simulink library "myLibrary"  (R2023b)
settings: Solver=VariableStepAuto  StartTime=0.0  StopTime=10.0  RelTol=1e-3
undefined symbols (not defined in the file): Cac_n1, ctrl1, Da, Discrete, dtha, ee_sli_rtmsupport, FA, gcbh, Ha, Ini, init_DCline, init_IPC, init_line, init_load, init_SG, init_shunt, init_TH, init_trafo, init_VSC, initMachineBlocks, Ka, Lf, Llkd_pu, Llkq1_pu, magnitude, NET, P, plots_step, q0, Rac_n1, Radd, Rkd_pu, Rkq1_pu, Rload_add, sim_config, sps_rtmsupport, spsSteamTurbineModel, T_DC_NET, T_global, T_IPC, T_load, T_NET, T_SG, T_shunt, T_STATCOM, T_TH, T_trafo, T_VSC, Ts, tstep, Udiff_a, V1
libraries: spsSeriesRLCBranchLib x105, eeGeneralControl x72, $bdroot x70, spsCurrentMeasurementLib x48, spsParallelRLCBranchLib x39, spsVoltageMeasurementLib x33, spsControlledVoltageSourceLib x27, spsFirstOrderFilterLib x16, dspsigops x6, spsThreePhaseVIMeasurementLib x5, spsPLL3phLib x4, spsThreePhaseBreakerLib x3
(part 9 of 12)

== system myLibrary/STATCOM/Control/Rotació ==
  V_q_diff : Inport
  V_d_diff : Inport  Port=2
  V_0_diff : Inport  Port=3
  Angle : Inport  Port=4
  Constant{2,5..7} (4 alike) : Constant  Value=0
  Constant8 : Constant
  Demux : Demux  Outputs=3
  Display : Display
  Gain1 : Gain  Gain=-1
  Matrix Concatenate : Concatenate  NumInputs=3  Mode=Multidimensional array  ConcatenateDimension=2
  Mux{,1..3} (4 alike) : Mux  Inputs=3
  Product : Product  Multiplication=Matrix(*)
  Trigonometric Function : Trigonometry  Operator=cos
  Trigonometric Function1 : Trigonometry
  Trigonometric Function2 : Trigonometry
  Trigonometric Function3 : Trigonometry  Operator=cos
  V_alfa_diff : Outport  VectorParamsAs1DForOutWhenUnconnected=off
  V_beta_diff : Outport  Port=2  VectorParamsAs1DForOutWhenUnconnected=off
  V_0 : Outport  Port=3  VectorParamsAs1DForOutWhenUnconnected=off
  wires:
  Angle/1 -> Trigonometric Function1/1, Trigonometric Function2/1, Trigonometric Function3/1, Trigonometric Function/1
  Trigonometric Function2/1 -> Mux2/1
  Gain1/1 -> Mux1/2
  Trigonometric Function/1 -> Mux1/1
  V_0_diff/1 -> Mux/3
  V_d_diff/1 -> Mux/2
  V_q_diff/1 -> Mux/1
  Matrix Concatenate/1 -> Product/1, Display/1
  Mux/1 -> Product/2
  Demux/3 -> V_0/1
  Demux/2 -> V_beta_diff/1
  Demux/1 -> V_alfa_diff/1
  Product/1 -> Demux/1
  Mux1/1 -> Matrix Concatenate/1
  Mux3/1 -> Matrix Concatenate/3
  Mux2/1 -> Matrix Concatenate/2
  Constant8/1 -> Mux3/3
  Constant7/1 -> Mux3/2
  Constant6/1 -> Mux3/1
  Constant5/1 -> Mux2/3
  Trigonometric Function3/1 -> Mux2/2
  Constant2/1 -> Mux1/3
  Trigonometric Function1/1 -> Gain1/1

== system myLibrary/STATCOM/Control/Subsystem ==
  Uq : Inport
  Ud : Inport  Port=2
  iq : Inport  Port=3
  id : Inport  Port=4
  Gain2 : Gain  Gain=3/2
  Product : Product
  Product1 : Product
  Sum8 : Sum
  Pac : Outport
  wires:
  Uq/1 -> Product/1
  Product/1 -> Sum8/1
  iq/1 -> Product/2
  id/1 -> Product1/2
  Gain2/1 -> Pac/1
  Ud/1 -> Product1/1
  Product1/1 -> Sum8/2
  Sum8/1 -> Gain2/1

== system myLibrary/qd transform/qd0 Transformation/Matriu T ==
  u : Inport
  Constant : Constant  Value=(2/3)*[1/2 1/2 1/2]
  Fcn : Fcn  Expr=(2/3)*cos(u)
  Fcn1 : Fcn  Expr=(2/3)*cos(u-(2*pi)/3)
  Fcn2 : Fcn  Expr=(2/3)*cos(u+(2*pi)/3)
  Fcn3 : Fcn  Expr=(2/3)*sin(u)
  Fcn4 : Fcn  Expr=(2/3)*sin(u-(2*pi)/3)
  Fcn5 : Fcn  Expr=(2/3)*sin(u+(2*pi)/3)
  Math Function : Math  Operator=transpose  SignedPower=on
  Matrix Concatenate : Concatenate  NumInputs=3  Mode=Multidimensional array  ConcatenateDimension=2
  Mux : Mux  Inputs=3
  Mux1 : Mux  Inputs=3
  Out1 : Outport  VectorParamsAs1DForOutWhenUnconnected=off
  wires:
  u/1 -> Fcn/1, Fcn1/1, Fcn2/1, Fcn3/1, Fcn4/1, Fcn5/1
  Fcn3/1 -> Mux1/1
  Fcn4/1 -> Mux1/2
  Fcn5/1 -> Mux1/3
  Mux/1 -> Matrix Concatenate/1
  Constant/1 -> Matrix Concatenate/3
  Fcn/1 -> Mux/1
  Fcn1/1 -> Mux/2
  Fcn2/1 -> Mux/3
  Mux1/1 -> Matrix Concatenate/2
  Matrix Concatenate/1 -> Math Function/1
  Math Function/1 -> Out1/1

== system myLibrary/AC-GFOL_DC-GFOL/Control Pac2/Is/Matriu T ==
  u : Inport
  Constant : Constant  Value=(2/3)*[1/2 1/2 1/2]
  Fcn : Fcn  Expr=(2/3)*cos(u)
  Fcn1 : Fcn  Expr=(2/3)*cos(u-(2*pi)/3)
  Fcn2 : Fcn  Expr=(2/3)*cos(u+(2*pi)/3)
  Fcn3 : Fcn  Expr=(2/3)*sin(u)
  Fcn4 : Fcn  Expr=(2/3)*sin(u-(2*pi)/3)
  Fcn5 : Fcn  Expr=(2/3)*sin(u+(2*pi)/3)
  Math Function : Math  Operator=transpose  SignedPower=on
  Matrix Concatenate : Concatenate  NumInputs=3  Mode=Multidimensional array  ConcatenateDimension=2
  Mux : Mux  Inputs=3
  Mux1 : Mux  Inputs=3
  Out1 : Outport  VectorParamsAs1DForOutWhenUnconnected=off
  wires:
  u/1 -> Fcn/1, Fcn1/1, Fcn2/1, Fcn3/1, Fcn4/1, Fcn5/1
  Fcn3/1 -> Mux1/1
  Fcn4/1 -> Mux1/2
  Fcn5/1 -> Mux1/3
  Mux/1 -> Matrix Concatenate/1
  Constant/1 -> Matrix Concatenate/3
  Fcn/1 -> Mux/1
  Fcn1/1 -> Mux/2
  Fcn2/1 -> Mux/3
  Mux1/1 -> Matrix Concatenate/2
  Matrix Concatenate/1 -> Math Function/1
  Math Function/1 -> Out1/1

== system myLibrary/AC-GFOL_DC-GFOL/Control Pac2/Is2/Matriu T ==
  u : Inport
  Constant : Constant  Value=(2/3)*[1/2 1/2 1/2]
  Fcn : Fcn  Expr=(2/3)*cos(u)
  Fcn1 : Fcn  Expr=(2/3)*cos(u-(2*pi)/3)
  Fcn2 : Fcn  Expr=(2/3)*cos(u+(2*pi)/3)
  Fcn3 : Fcn  Expr=(2/3)*sin(u)
  Fcn4 : Fcn  Expr=(2/3)*sin(u-(2*pi)/3)
  Fcn5 : Fcn  Expr=(2/3)*sin(u+(2*pi)/3)
  Math Function : Math  Operator=transpose  SignedPower=on
  Matrix Concatenate : Concatenate  NumInputs=3  Mode=Multidimensional array  ConcatenateDimension=2
  Mux : Mux  Inputs=3
  Mux1 : Mux  Inputs=3
  Out1 : Outport  VectorParamsAs1DForOutWhenUnconnected=off
  wires:
  u/1 -> Fcn/1, Fcn1/1, Fcn2/1, Fcn3/1, Fcn4/1, Fcn5/1
  Fcn3/1 -> Mux1/1
  Fcn4/1 -> Mux1/2
  Fcn5/1 -> Mux1/3
  Mux/1 -> Matrix Concatenate/1
  Constant/1 -> Matrix Concatenate/3
  Fcn/1 -> Mux/1
  Fcn1/1 -> Mux/2
  Fcn2/1 -> Mux/3
  Mux1/1 -> Matrix Concatenate/2
  Matrix Concatenate/1 -> Math Function/1
  Math Function/1 -> Out1/1

== system myLibrary/AC-GFOL_DC-GFOL/Control Pac2/l_DC_alfa//beta/Clarke ==
  Isum : Inport
  Constant : Constant
  Constant1 : Constant  Value=-1/2
  Constant2 : Constant  Value=-1/2
  Constant3 : Constant  Value=0
  Constant4 : Constant  Value=-sqrt(3)/2
  Constant5 : Constant  Value=sqrt(3)/2
  Constant6 : Constant  Value=1/2
  Constant7 : Constant  Value=1/2
  Constant8 : Constant  Value=1/2
  Demux : Demux  Outputs=3
  Display : Display
  Gain : Gain  Gain=2/3
  Math Function : Math  Operator=transpose  SignedPower=on
  Matrix Concatenate : Concatenate  NumInputs=3  Mode=Multidimensional array  ConcatenateDimension=2
  Mux1 : Mux  Inputs=3
  Mux2 : Mux  Inputs=3
  Mux3 : Mux  Inputs=3
  Product : Product  Multiplication=Matrix(*)
  I_alfa : Outport  VectorParamsAs1DForOutWhenUnconnected=off
  I_beta : Outport  Port=2  VectorParamsAs1DForOutWhenUnconnected=off
  I_0 : Outport  Port=3  VectorParamsAs1DForOutWhenUnconnected=off
  wires:
  Constant/1 -> Mux1/1
  Constant1/1 -> Mux1/2
  Constant2/1 -> Mux1/3
  Constant3/1 -> Mux2/1
  Constant4/1 -> Mux2/2
  Constant5/1 -> Mux2/3
  Constant6/1 -> Mux3/1
  Constant7/1 -> Mux3/2
  Constant8/1 -> Mux3/3
  Math Function/1 -> Gain/1
  Matrix Concatenate/1 -> Math Function/1
  Mux2/1 -> Matrix Concatenate/2
  Mux3/1 -> Matrix Concatenate/3
  Mux1/1 -> Matrix Concatenate/1
  Product/1 -> Demux/1
  Demux/1 -> I_alfa/1
  Demux/2 -> I_beta/1
  Demux/3 -> I_0/1
  Gain/1 -> Display/1, Product/1
  Isum/1 -> Product/2

== system myLibrary/AC-GFOL_DC-GFOR/Control Pac2/Is/Matriu T ==
  u : Inport
  Constant : Constant  Value=(2/3)*[1/2 1/2 1/2]
  Fcn : Fcn  Expr=(2/3)*cos(u)
  Fcn1 : Fcn  Expr=(2/3)*cos(u-(2*pi)/3)
  Fcn2 : Fcn  Expr=(2/3)*cos(u+(2*pi)/3)
  Fcn3 : Fcn  Expr=(2/3)*sin(u)
  Fcn4 : Fcn  Expr=(2/3)*sin(u-(2*pi)/3)
  Fcn5 : Fcn  Expr=(2/3)*sin(u+(2*pi)/3)
  Math Function : Math  Operator=transpose  SignedPower=on
  Matrix Concatenate : Concatenate  NumInputs=3  Mode=Multidimensional array  ConcatenateDimension=2
  Mux : Mux  Inputs=3
  Mux1 : Mux  Inputs=3
  Out1 : Outport  VectorParamsAs1DForOutWhenUnconnected=off
  wires:
  u/1 -> Fcn/1, Fcn1/1, Fcn2/1, Fcn3/1, Fcn4/1, Fcn5/1
  Fcn3/1 -> Mux1/1
  Fcn4/1 -> Mux1/2
  Fcn5/1 -> Mux1/3
  Mux/1 -> Matrix Concatenate/1
  Constant/1 -> Matrix Concatenate/3
  Fcn/1 -> Mux/1
  Fcn1/1 -> Mux/2
  Fcn2/1 -> Mux/3
  Mux1/1 -> Matrix Concatenate/2
  Matrix Concatenate/1 -> Math Function/1
  Math Function/1 -> Out1/1

== system myLibrary/AC-GFOL_DC-GFOR/Control Pac2/Is2/Matriu T ==
  u : Inport
  Constant : Constant  Value=(2/3)*[1/2 1/2 1/2]
  Fcn : Fcn  Expr=(2/3)*cos(u)
  Fcn1 : Fcn  Expr=(2/3)*cos(u-(2*pi)/3)
  Fcn2 : Fcn  Expr=(2/3)*cos(u+(2*pi)/3)
  Fcn3 : Fcn  Expr=(2/3)*sin(u)
  Fcn4 : Fcn  Expr=(2/3)*sin(u-(2*pi)/3)
  Fcn5 : Fcn  Expr=(2/3)*sin(u+(2*pi)/3)
  Math Function : Math  Operator=transpose  SignedPower=on
  Matrix Concatenate : Concatenate  NumInputs=3  Mode=Multidimensional array  ConcatenateDimension=2
  Mux : Mux  Inputs=3
  Mux1 : Mux  Inputs=3
  Out1 : Outport  VectorParamsAs1DForOutWhenUnconnected=off
  wires:
  u/1 -> Fcn/1, Fcn1/1, Fcn2/1, Fcn3/1, Fcn4/1, Fcn5/1
  Fcn3/1 -> Mux1/1
  Fcn4/1 -> Mux1/2
  Fcn5/1 -> Mux1/3
  Mux/1 -> Matrix Concatenate/1
  Constant/1 -> Matrix Concatenate/3
  Fcn/1 -> Mux/1
  Fcn1/1 -> Mux/2
  Fcn2/1 -> Mux/3
  Mux1/1 -> Matrix Concatenate/2
  Matrix Concatenate/1 -> Math Function/1
  Math Function/1 -> Out1/1

== system myLibrary/AC-GFOL_DC-GFOR/Control Pac2/l_DC_alfa//beta/Clarke ==
  Isum : Inport
  Constant : Constant
  Constant1 : Constant  Value=-1/2
  Constant2 : Constant  Value=-1/2
  Constant3 : Constant  Value=0
  Constant4 : Constant  Value=-sqrt(3)/2
  Constant5 : Constant  Value=sqrt(3)/2
  Constant6 : Constant  Value=1/2
  Constant7 : Constant  Value=1/2
  Constant8 : Constant  Value=1/2
  Demux : Demux  Outputs=3
  Display : Display
  Gain : Gain  Gain=2/3
  Math Function : Math  Operator=transpose  SignedPower=on
  Matrix Concatenate : Concatenate  NumInputs=3  Mode=Multidimensional array  ConcatenateDimension=2
  Mux1 : Mux  Inputs=3
  Mux2 : Mux  Inputs=3
  Mux3 : Mux  Inputs=3
  Product : Product  Multiplication=Matrix(*)
  I_alfa : Outport  VectorParamsAs1DForOutWhenUnconnected=off
  I_beta : Outport  Port=2  VectorParamsAs1DForOutWhenUnconnected=off
  I_0 : Outport  Port=3  VectorParamsAs1DForOutWhenUnconnected=off
  wires:
  Constant/1 -> Mux1/1
  Constant1/1 -> Mux1/2
  Constant2/1 -> Mux1/3
  Constant3/1 -> Mux2/1
  Constant4/1 -> Mux2/2
  Constant5/1 -> Mux2/3
  Constant6/1 -> Mux3/1
  Constant7/1 -> Mux3/2
  Constant8/1 -> Mux3/3
  Math Function/1 -> Gain/1
  Matrix Concatenate/1 -> Math Function/1
  Mux2/1 -> Matrix Concatenate/2
  Mux3/1 -> Matrix Concatenate/3
  Mux1/1 -> Matrix Concatenate/1
  Product/1 -> Demux/1
  Demux/1 -> I_alfa/1
  Demux/2 -> I_beta/1
  Demux/3 -> I_0/1
  Gain/1 -> Display/1, Product/1
  Isum/1 -> Product/2

== system myLibrary/AC-GFOR_DC-GFOL/Control Pac2/Is/Matriu T ==
  u : Inport
  Constant : Constant  Value=(2/3)*[1/2 1/2 1/2]
  Fcn : Fcn  Expr=(2/3)*cos(u)
  Fcn1 : Fcn  Expr=(2/3)*cos(u-(2*pi)/3)
  Fcn2 : Fcn  Expr=(2/3)*cos(u+(2*pi)/3)
  Fcn3 : Fcn  Expr=(2/3)*sin(u)
  Fcn4 : Fcn  Expr=(2/3)*sin(u-(2*pi)/3)
  Fcn5 : Fcn  Expr=(2/3)*sin(u+(2*pi)/3)
  Math Function : Math  Operator=transpose  SignedPower=on
  Matrix Concatenate : Concatenate  NumInputs=3  Mode=Multidimensional array  ConcatenateDimension=2
  Mux : Mux  Inputs=3
  Mux1 : Mux  Inputs=3
  Out1 : Outport  VectorParamsAs1DForOutWhenUnconnected=off
  wires:
  Math Function/1 -> Out1/1
  Matrix Concatenate/1 -> Math Function/1
  Mux1/1 -> Matrix Concatenate/2
  Fcn2/1 -> Mux/3
  Fcn1/1 -> Mux/2
  Fcn/1 -> Mux/1
  Constant/1 -> Matrix Concatenate/3
  Mux/1 -> Matrix Concatenate/1
  Fcn5/1 -> Mux1/3
  Fcn4/1 -> Mux1/2
  Fcn3/1 -> Mux1/1
  u/1 -> Fcn5/1, Fcn4/1, Fcn3/1, Fcn2/1, Fcn1/1, Fcn/1

== system myLibrary/AC-GFOR_DC-GFOL/Control Pac2/Is2/Matriu T ==
  u : Inport
  Constant : Constant  Value=(2/3)*[1/2 1/2 1/2]
  Fcn : Fcn  Expr=(2/3)*cos(u)
  Fcn1 : Fcn  Expr=(2/3)*cos(u-(2*pi)/3)
  Fcn2 : Fcn  Expr=(2/3)*cos(u+(2*pi)/3)
  Fcn3 : Fcn  Expr=(2/3)*sin(u)
  Fcn4 : Fcn  Expr=(2/3)*sin(u-(2*pi)/3)
  Fcn5 : Fcn  Expr=(2/3)*sin(u+(2*pi)/3)
  Math Function : Math  Operator=transpose  SignedPower=on
  Matrix Concatenate : Concatenate  NumInputs=3  Mode=Multidimensional array  ConcatenateDimension=2
  Mux : Mux  Inputs=3
  Mux1 : Mux  Inputs=3
  Out1 : Outport  VectorParamsAs1DForOutWhenUnconnected=off
  wires:
  Math Function/1 -> Out1/1
  Matrix Concatenate/1 -> Math Function/1
  Mux1/1 -> Matrix Concatenate/2
  Fcn2/1 -> Mux/3
  Fcn1/1 -> Mux/2
  Fcn/1 -> Mux/1
  Constant/1 -> Matrix Concatenate/3
  Mux/1 -> Matrix Concatenate/1
  Fcn5/1 -> Mux1/3
  Fcn4/1 -> Mux1/2
  Fcn3/1 -> Mux1/1
  u/1 -> Fcn5/1, Fcn4/1, Fcn3/1, Fcn2/1, Fcn1/1, Fcn/1

== system myLibrary/AC-GFOR_DC-GFOL/Control Pac2/l_DC_alfa//beta/Clarke ==
  Isum : Inport
  Constant : Constant
  Constant1 : Constant  Value=-1/2
  Constant2 : Constant  Value=-1/2
  Constant3 : Constant  Value=0
  Constant4 : Constant  Value=-sqrt(3)/2
  Constant5 : Constant  Value=sqrt(3)/2
  Constant6 : Constant  Value=1/2
  Constant7 : Constant  Value=1/2
  Constant8 : Constant  Value=1/2
  Demux : Demux  Outputs=3
  Display : Display
  Gain : Gain  Gain=2/3
  Math Function : Math  Operator=transpose  SignedPower=on
  Matrix Concatenate : Concatenate  NumInputs=3  Mode=Multidimensional array  ConcatenateDimension=2
  Mux1 : Mux  Inputs=3
  Mux2 : Mux  Inputs=3
  Mux3 : Mux  Inputs=3
  Product : Product  Multiplication=Matrix(*)
  I_alfa : Outport  VectorParamsAs1DForOutWhenUnconnected=off
  I_beta : Outport  Port=2  VectorParamsAs1DForOutWhenUnconnected=off
  I_0 : Outport  Port=3  VectorParamsAs1DForOutWhenUnconnected=off
  wires:
  Isum/1 -> Product/2
  Gain/1 -> Product/1, Display/1
  Demux/3 -> I_0/1
  Demux/2 -> I_beta/1
  Demux/1 -> I_alfa/1
  Product/1 -> Demux/1
  Mux1/1 -> Matrix Concatenate/1
  Mux3/1 -> Matrix Concatenate/3
  Mux2/1 -> Matrix Concatenate/2
  Matrix Concatenate/1 -> Math Function/1
  Math Function/1 -> Gain/1
  Constant8/1 -> Mux3/3
  Constant7/1 -> Mux3/2
  Constant6/1 -> Mux3/1
  Constant5/1 -> Mux2/3
  Constant4/1 -> Mux2/2
  Constant3/1 -> Mux2/1
  Constant2/1 -> Mux1/3
  Constant1/1 -> Mux1/2
  Constant/1 -> Mux1/1

== system myLibrary/GFOL/Control/Is/Matriu T ==
  u : Inport
  Constant : Constant  Value=(2/3)*[1/2 1/2 1/2]
  Fcn : Fcn  Expr=(2/3)*cos(u)
  Fcn1 : Fcn  Expr=(2/3)*cos(u-(2*pi)/3)
  Fcn2 : Fcn  Expr=(2/3)*cos(u+(2*pi)/3)
  Fcn3 : Fcn  Expr=(2/3)*sin(u)
  Fcn4 : Fcn  Expr=(2/3)*sin(u-(2*pi)/3)
  Fcn5 : Fcn  Expr=(2/3)*sin(u+(2*pi)/3)
  Math Function : Math  Operator=transpose  SignedPower=on
  Matrix Concatenate : Concatenate  NumInputs=3  Mode=Multidimensional array  ConcatenateDimension=2
  Mux : Mux  Inputs=3
  Mux1 : Mux  Inputs=3
  Out1 : Outport  VectorParamsAs1DForOutWhenUnconnected=off
  wires:
  u/1 -> Fcn/1, Fcn1/1, Fcn2/1, Fcn3/1, Fcn4/1, Fcn5/1
  Fcn3/1 -> Mux1/1
  Fcn4/1 -> Mux1/2
  Fcn5/1 -> Mux1/3
  Mux/1 -> Matrix Concatenate/1
  Constant/1 -> Matrix Concatenate/3
  Fcn/1 -> Mux/1
  Fcn1/1 -> Mux/2
  Fcn2/1 -> Mux/3
  Mux1/1 -> Matrix Concatenate/2
  Matrix Concatenate/1 -> Math Function/1
  Math Function/1 -> Out1/1

== system myLibrary/GFOL/Control/Is1/Matriu T ==
  u : Inport
  Constant : Constant  Value=(2/3)*[1/2 1/2 1/2]
  Fcn : Fcn  Expr=(2/3)*cos(u)
  Fcn1 : Fcn  Expr=(2/3)*cos(u-(2*pi)/3)
  Fcn2 : Fcn  Expr=(2/3)*cos(u+(2*pi)/3)
  Fcn3 : Fcn  Expr=(2/3)*sin(u)
  Fcn4 : Fcn  Expr=(2/3)*sin(u-(2*pi)/3)
  Fcn5 : Fcn  Expr=(2/3)*sin(u+(2*pi)/3)
  Math Function : Math  Operator=transpose  SignedPower=on
  Matrix Concatenate : Concatenate  NumInputs=3  Mode=Multidimensional array  ConcatenateDimension=2
  Mux : Mux  Inputs=3
  Mux1 : Mux  Inputs=3
  Out1 : Outport  VectorParamsAs1DForOutWhenUnconnected=off
  wires:
  Math Function/1 -> Out1/1
  Matrix Concatenate/1 -> Math Function/1
  Mux1/1 -> Matrix Concatenate/2
  Fcn2/1 -> Mux/3
  Fcn1/1 -> Mux/2
  Fcn/1 -> Mux/1
  Constant/1 -> Matrix Concatenate/3
  Mux/1 -> Matrix Concatenate/1
  Fcn5/1 -> Mux1/3
  Fcn4/1 -> Mux1/2
  Fcn3/1 -> Mux1/1
  u/1 -> Fcn5/1, Fcn4/1, Fcn3/1, Fcn2/1, Fcn1/1, Fcn/1

== system myLibrary/GFOL/Control/Is3/Matriu T ==
  u : Inport
  Constant : Constant  Value=(2/3)*[1/2 1/2 1/2]
  Fcn : Fcn  Expr=(2/3)*cos(u)
  Fcn1 : Fcn  Expr=(2/3)*cos(u-(2*pi)/3)
  Fcn2 : Fcn  Expr=(2/3)*cos(u+(2*pi)/3)
  Fcn3 : Fcn  Expr=(2/3)*sin(u)
  Fcn4 : Fcn  Expr=(2/3)*sin(u-(2*pi)/3)
  Fcn5 : Fcn  Expr=(2/3)*sin(u+(2*pi)/3)
  Math Function : Math  Operator=transpose  SignedPower=on
  Matrix Concatenate : Concatenate  NumInputs=3  Mode=Multidimensional array  ConcatenateDimension=2
  Mux : Mux  Inputs=3
  Mux1 : Mux  Inputs=3
  Out1 : Outport  VectorParamsAs1DForOutWhenUnconnected=off
  wires:
  u/1 -> Fcn/1, Fcn1/1, Fcn2/1, Fcn3/1, Fcn4/1, Fcn5/1
  Fcn3/1 -> Mux1/1
  Fcn4/1 -> Mux1/2
  Fcn5/1 -> Mux1/3
  Mux/1 -> Matrix Concatenate/1
  Constant/1 -> Matrix Concatenate/3
  Fcn/1 -> Mux/1
  Fcn1/1 -> Mux/2
  Fcn2/1 -> Mux/3
  Mux1/1 -> Matrix Concatenate/2
  Matrix Concatenate/1 -> Math Function/1
  Math Function/1 -> Out1/1

== system myLibrary/GFOL/Control/Is4/Matriu T ==
  u : Inport
  Constant : Constant  Value=(2/3)*[1/2 1/2 1/2]
  Fcn : Fcn  Expr=(2/3)*cos(u)
  Fcn1 : Fcn  Expr=(2/3)*cos(u-(2*pi)/3)
  Fcn2 : Fcn  Expr=(2/3)*cos(u+(2*pi)/3)
  Fcn3 : Fcn  Expr=(2/3)*sin(u)
  Fcn4 : Fcn  Expr=(2/3)*sin(u-(2*pi)/3)
  Fcn5 : Fcn  Expr=(2/3)*sin(u+(2*pi)/3)
  Math Function : Math  Operator=transpose  SignedPower=on
  Matrix Concatenate : Concatenate  NumInputs=3  Mode=Multidimensional array  ConcatenateDimension=2
  Mux : Mux  Inputs=3
  Mux1 : Mux  Inputs=3
  Out1 : Outport  VectorParamsAs1DForOutWhenUnconnected=off
  wires:
  Math Function/1 -> Out1/1
  Matrix Concatenate/1 -> Math Function/1
  Mux1/1 -> Matrix Concatenate/2
  Fcn2/1 -> Mux/3
  Fcn1/1 -> Mux/2
  Fcn/1 -> Mux/1
  Constant/1 -> Matrix Concatenate/3
  Mux/1 -> Matrix Concatenate/1
  Fcn5/1 -> Mux1/3
  Fcn4/1 -> Mux1/2
  Fcn3/1 -> Mux1/1
  u/1 -> Fcn5/1, Fcn4/1, Fcn3/1, Fcn2/1, Fcn1/1, Fcn/1

== system myLibrary/GFOL/Control/Is5/Matriu T ==
  u : Inport
  Constant : Constant  Value=(2/3)*[1/2 1/2 1/2]
  Fcn : Fcn  Expr=(2/3)*cos(u)
  Fcn1 : Fcn  Expr=(2/3)*cos(u-(2*pi)/3)
  Fcn2 : Fcn  Expr=(2/3)*cos(u+(2*pi)/3)
  Fcn3 : Fcn  Expr=(2/3)*sin(u)
  Fcn4 : Fcn  Expr=(2/3)*sin(u-(2*pi)/3)
  Fcn5 : Fcn  Expr=(2/3)*sin(u+(2*pi)/3)
  Math Function : Math  Operator=transpose  SignedPower=on
  Matrix Concatenate : Concatenate  NumInputs=3  Mode=Multidimensional array  ConcatenateDimension=2
  Mux : Mux  Inputs=3
  Mux1 : Mux  Inputs=3
  Out1 : Outport  VectorParamsAs1DForOutWhenUnconnected=off
  wires:
  u/1 -> Fcn/1, Fcn1/1, Fcn2/1, Fcn3/1, Fcn4/1, Fcn5/1
  Fcn3/1 -> Mux1/1
  Fcn4/1 -> Mux1/2
  Fcn5/1 -> Mux1/3
  Mux/1 -> Matrix Concatenate/1
  Constant/1 -> Matrix Concatenate/3
  Fcn/1 -> Mux/1
  Fcn1/1 -> Mux/2
  Fcn2/1 -> Mux/3
  Mux1/1 -> Matrix Concatenate/2
  Matrix Concatenate/1 -> Math Function/1
  Math Function/1 -> Out1/1

== system myLibrary/GFOL/Control/Is7/Matriu T ==
  u : Inport
  Constant : Constant  Value=(2/3)*[1/2 1/2 1/2]
  Fcn : Fcn  Expr=(2/3)*cos(u)
  Fcn1 : Fcn  Expr=(2/3)*cos(u-(2*pi)/3)
  Fcn2 : Fcn  Expr=(2/3)*cos(u+(2*pi)/3)
  Fcn3 : Fcn  Expr=(2/3)*sin(u)
  Fcn4 : Fcn  Expr=(2/3)*sin(u-(2*pi)/3)
  Fcn5 : Fcn  Expr=(2/3)*sin(u+(2*pi)/3)
  Math Function : Math  Operator=transpose  SignedPower=on
  Matrix Concatenate : Concatenate  NumInputs=3  Mode=Multidimensional array  ConcatenateDimension=2
  Mux : Mux  Inputs=3
  Mux1 : Mux  Inputs=3
  Out1 : Outport  VectorParamsAs1DForOutWhenUnconnected=off
  wires:
  Math Function/1 -> Out1/1
  Matrix Concatenate/1 -> Math Function/1
  Mux1/1 -> Matrix Concatenate/2
  Fcn2/1 -> Mux/3
  Fcn1/1 -> Mux/2
  Fcn/1 -> Mux/1
  Constant/1 -> Matrix Concatenate/3
  Mux/1 -> Matrix Concatenate/1
  Fcn5/1 -> Mux1/3
  Fcn4/1 -> Mux1/2
  Fcn3/1 -> Mux1/1
  u/1 -> Fcn5/1, Fcn4/1, Fcn3/1, Fcn2/1, Fcn1/1, Fcn/1

== system myLibrary/GFOL/Control/PLL/Tpark ==
  Va : Inport
  Vb : Inport  Port=2
  Vc : Inport  Port=3
  u : Inport  Port=4
  Demux : Demux  Outputs=3
  Matriu T : Subsystem
  Mux : Mux  Inputs=3
      settings: DisplayOption=signals
  Product : Product  Multiplication=Matrix(*)
  Vq : Outport  VectorParamsAs1DForOutWhenUnconnected=off
  Vd : Outport  Port=2  VectorParamsAs1DForOutWhenUnconnected=off
  0 : Outport  Port=3  VectorParamsAs1DForOutWhenUnconnected=off
  wires:
  Matriu T/1(Out1) -> Product/1
  Mux/1 -> Product/2
  u/1 -> Matriu T/1(u)
  Demux/3 -> 0/1
  Demux/2 -> Vd/1
  Demux/1 -> Vq/1
  Product/1 -> Demux/1
  Vc/1 -> Mux/3
  Vb/1 -> Mux/2
  Va/1 -> Mux/1

== system myLibrary/GFOL_RL/Control/Is/Matriu T ==
  u : Inport
  Constant : Constant  Value=(2/3)*[1/2 1/2 1/2]
  Fcn : Fcn  Expr=(2/3)*cos(u)
  Fcn1 : Fcn  Expr=(2/3)*cos(u-(2*pi)/3)
  Fcn2 : Fcn  Expr=(2/3)*cos(u+(2*pi)/3)
  Fcn3 : Fcn  Expr=(2/3)*sin(u)
  Fcn4 : Fcn  Expr=(2/3)*sin(u-(2*pi)/3)
  Fcn5 : Fcn  Expr=(2/3)*sin(u+(2*pi)/3)
  Math Function : Math  Operator=transpose  SignedPower=on
  Matrix Concatenate : Concatenate  NumInputs=3  Mode=Multidimensional array  ConcatenateDimension=2
  Mux : Mux  Inputs=3
  Mux1 : Mux  Inputs=3
  Out1 : Outport  VectorParamsAs1DForOutWhenUnconnected=off
  wires:
  u/1 -> Fcn/1, Fcn1/1, Fcn2/1, Fcn3/1, Fcn4/1, Fcn5/1
  Fcn3/1 -> Mux1/1
  Fcn4/1 -> Mux1/2
  Fcn5/1 -> Mux1/3
  Mux/1 -> Matrix Concatenate/1
  Constant/1 -> Matrix Concatenate/3
  Fcn/1 -> Mux/1
  Fcn1/1 -> Mux/2
  Fcn2/1 -> Mux/3
  Mux1/1 -> Matrix Concatenate/2
  Matrix Concatenate/1 -> Math Function/1
  Math Function/1 -> Out1/1

== system myLibrary/GFOL_RL/Control/Is1/Matriu T ==
  u : Inport
  Constant : Constant  Value=(2/3)*[1/2 1/2 1/2]
  Fcn : Fcn  Expr=(2/3)*cos(u)
  Fcn1 : Fcn  Expr=(2/3)*cos(u-(2*pi)/3)
  Fcn2 : Fcn  Expr=(2/3)*cos(u+(2*pi)/3)
  Fcn3 : Fcn  Expr=(2/3)*sin(u)
  Fcn4 : Fcn  Expr=(2/3)*sin(u-(2*pi)/3)
  Fcn5 : Fcn  Expr=(2/3)*sin(u+(2*pi)/3)
  Math Function : Math  Operator=transpose  SignedPower=on
  Matrix Concatenate : Concatenate  NumInputs=3  Mode=Multidimensional array  ConcatenateDimension=2
  Mux : Mux  Inputs=3
  Mux1 : Mux  Inputs=3
  Out1 : Outport  VectorParamsAs1DForOutWhenUnconnected=off
  wires:
  Math Function/1 -> Out1/1
  Matrix Concatenate/1 -> Math Function/1
  Mux1/1 -> Matrix Concatenate/2
  Fcn2/1 -> Mux/3
  Fcn1/1 -> Mux/2
  Fcn/1 -> Mux/1
  Constant/1 -> Matrix Concatenate/3
  Mux/1 -> Matrix Concatenate/1
  Fcn5/1 -> Mux1/3
  Fcn4/1 -> Mux1/2
  Fcn3/1 -> Mux1/1
  u/1 -> Fcn5/1, Fcn4/1, Fcn3/1, Fcn2/1, Fcn1/1, Fcn/1

== system myLibrary/GFOL_RL/Control/Is3/Matriu T ==
  u : Inport
  Constant : Constant  Value=(2/3)*[1/2 1/2 1/2]
  Fcn : Fcn  Expr=(2/3)*cos(u)
  Fcn1 : Fcn  Expr=(2/3)*cos(u-(2*pi)/3)
  Fcn2 : Fcn  Expr=(2/3)*cos(u+(2*pi)/3)
  Fcn3 : Fcn  Expr=(2/3)*sin(u)
  Fcn4 : Fcn  Expr=(2/3)*sin(u-(2*pi)/3)
  Fcn5 : Fcn  Expr=(2/3)*sin(u+(2*pi)/3)
  Math Function : Math  Operator=transpose  SignedPower=on
  Matrix Concatenate : Concatenate  NumInputs=3  Mode=Multidimensional array  ConcatenateDimension=2
  Mux : Mux  Inputs=3
  Mux1 : Mux  Inputs=3
  Out1 : Outport  VectorParamsAs1DForOutWhenUnconnected=off
  wires:
  u/1 -> Fcn/1, Fcn1/1, Fcn2/1, Fcn3/1, Fcn4/1, Fcn5/1
  Fcn3/1 -> Mux1/1
  Fcn4/1 -> Mux1/2
  Fcn5/1 -> Mux1/3
  Mux/1 -> Matrix Concatenate/1
  Constant/1 -> Matrix Concatenate/3
  Fcn/1 -> Mux/1
  Fcn1/1 -> Mux/2
  Fcn2/1 -> Mux/3
  Mux1/1 -> Matrix Concatenate/2
  Matrix Concatenate/1 -> Math Function/1
  Math Function/1 -> Out1/1

== system myLibrary/GFOL_RL/Control/Is4/Matriu T ==
  u : Inport
  Constant : Constant  Value=(2/3)*[1/2 1/2 1/2]
  Fcn : Fcn  Expr=(2/3)*cos(u)
  Fcn1 : Fcn  Expr=(2/3)*cos(u-(2*pi)/3)
  Fcn2 : Fcn  Expr=(2/3)*cos(u+(2*pi)/3)
  Fcn3 : Fcn  Expr=(2/3)*sin(u)
  Fcn4 : Fcn  Expr=(2/3)*sin(u-(2*pi)/3)
  Fcn5 : Fcn  Expr=(2/3)*sin(u+(2*pi)/3)
  Math Function : Math  Operator=transpose  SignedPower=on
  Matrix Concatenate : Concatenate  NumInputs=3  Mode=Multidimensional array  ConcatenateDimension=2
  Mux : Mux  Inputs=3
  Mux1 : Mux  Inputs=3
  Out1 : Outport  VectorParamsAs1DForOutWhenUnconnected=off
  wires:
  Math Function/1 -> Out1/1
  Matrix Concatenate/1 -> Math Function/1
  Mux1/1 -> Matrix Concatenate/2
  Fcn2/1 -> Mux/3
  Fcn1/1 -> Mux/2
  Fcn/1 -> Mux/1
  Constant/1 -> Matrix Concatenate/3
  Mux/1 -> Matrix Concatenate/1
  Fcn5/1 -> Mux1/3
  Fcn4/1 -> Mux1/2
  Fcn3/1 -> Mux1/1
  u/1 -> Fcn5/1, Fcn4/1, Fcn3/1, Fcn2/1, Fcn1/1, Fcn/1

== system myLibrary/GFOL_RL/Control/Is5/Matriu T ==
  u : Inport
  Constant : Constant  Value=(2/3)*[1/2 1/2 1/2]
  Fcn : Fcn  Expr=(2/3)*cos(u)
  Fcn1 : Fcn  Expr=(2/3)*cos(u-(2*pi)/3)
  Fcn2 : Fcn  Expr=(2/3)*cos(u+(2*pi)/3)
  Fcn3 : Fcn  Expr=(2/3)*sin(u)
  Fcn4 : Fcn  Expr=(2/3)*sin(u-(2*pi)/3)
  Fcn5 : Fcn  Expr=(2/3)*sin(u+(2*pi)/3)
  Math Function : Math  Operator=transpose  SignedPower=on
  Matrix Concatenate : Concatenate  NumInputs=3  Mode=Multidimensional array  ConcatenateDimension=2
  Mux : Mux  Inputs=3
  Mux1 : Mux  Inputs=3
  Out1 : Outport  VectorParamsAs1DForOutWhenUnconnected=off
  wires:
  u/1 -> Fcn/1, Fcn1/1, Fcn2/1, Fcn3/1, Fcn4/1, Fcn5/1
  Fcn3/1 -> Mux1/1
  Fcn4/1 -> Mux1/2
  Fcn5/1 -> Mux1/3
  Mux/1 -> Matrix Concatenate/1
  Constant/1 -> Matrix Concatenate/3
  Fcn/1 -> Mux/1
  Fcn1/1 -> Mux/2
  Fcn2/1 -> Mux/3
  Mux1/1 -> Matrix Concatenate/2
  Matrix Concatenate/1 -> Math Function/1
  Math Function/1 -> Out1/1

== system myLibrary/GFOL_RL/Control/PLL/Tpark ==
  Va : Inport
  Vb : Inport  Port=2
  Vc : Inport  Port=3
  u : Inport  Port=4
  Demux : Demux  Outputs=3
  Matriu T : Subsystem
  Mux : Mux  Inputs=3
      settings: DisplayOption=signals
  Product : Product  Multiplication=Matrix(*)
  Vq : Outport  VectorParamsAs1DForOutWhenUnconnected=off
  Vd : Outport  Port=2  VectorParamsAs1DForOutWhenUnconnected=off
  0 : Outport  Port=3  VectorParamsAs1DForOutWhenUnconnected=off
  wires:
  Matriu T/1(Out1) -> Product/1
  Mux/1 -> Product/2
  u/1 -> Matriu T/1(u)
  Demux/3 -> 0/1
  Demux/2 -> Vd/1
  Demux/1 -> Vq/1
  Product/1 -> Demux/1
  Vc/1 -> Mux/3
  Vb/1 -> Mux/2
  Va/1 -> Mux/1

== system myLibrary/GFOR/Control/Is/Matriu T ==
  u : Inport
  Constant : Constant  Value=(2/3)*[1/2 1/2 1/2]
  Fcn : Fcn  Expr=(2/3)*cos(u)
  Fcn1 : Fcn  Expr=(2/3)*cos(u-(2*pi)/3)
  Fcn2 : Fcn  Expr=(2/3)*cos(u+(2*pi)/3)
  Fcn3 : Fcn  Expr=(2/3)*sin(u)
  Fcn4 : Fcn  Expr=(2/3)*sin(u-(2*pi)/3)
  Fcn5 : Fcn  Expr=(2/3)*sin(u+(2*pi)/3)
  Math Function : Math  Operator=transpose  SignedPower=on
  Matrix Concatenate : Concatenate  NumInputs=3  Mode=Multidimensional array  ConcatenateDimension=2
  Mux : Mux  Inputs=3
  Mux1 : Mux  Inputs=3
  Out1 : Outport  VectorParamsAs1DForOutWhenUnconnected=off
  wires:
  Math Function/1 -> Out1/1
  Matrix Concatenate/1 -> Math Function/1
  Mux1/1 -> Matrix Concatenate/2
  Fcn2/1 -> Mux/3
  Fcn1/1 -> Mux/2
  Fcn/1 -> Mux/1
  Constant/1 -> Matrix Concatenate/3
  Mux/1 -> Matrix Concatenate/1
  Fcn5/1 -> Mux1/3
  Fcn4/1 -> Mux1/2
  Fcn3/1 -> Mux1/1
  u/1 -> Fcn5/1, Fcn4/1, Fcn3/1, Fcn2/1, Fcn1/1, Fcn/1

== system myLibrary/GFOR/Control/Is2/Matriu T ==
  u : Inport
  Constant : Constant  Value=(2/3)*[1/2 1/2 1/2]
  Fcn : Fcn  Expr=(2/3)*cos(u)
  Fcn1 : Fcn  Expr=(2/3)*cos(u-(2*pi)/3)
  Fcn2 : Fcn  Expr=(2/3)*cos(u+(2*pi)/3)
  Fcn3 : Fcn  Expr=(2/3)*sin(u)
  Fcn4 : Fcn  Expr=(2/3)*sin(u-(2*pi)/3)
  Fcn5 : Fcn  Expr=(2/3)*sin(u+(2*pi)/3)
  Math Function : Math  Operator=transpose  SignedPower=on
  Matrix Concatenate : Concatenate  NumInputs=3  Mode=Multidimensional array  ConcatenateDimension=2
  Mux : Mux  Inputs=3
  Mux1 : Mux  Inputs=3
  Out1 : Outport  VectorParamsAs1DForOutWhenUnconnected=off
  wires:
  Math Function/1 -> Out1/1
  Matrix Concatenate/1 -> Math Function/1
  Mux1/1 -> Matrix Concatenate/2
  Fcn2/1 -> Mux/3
  Fcn1/1 -> Mux/2
  Fcn/1 -> Mux/1
  Constant/1 -> Matrix Concatenate/3
  Mux/1 -> Matrix Concatenate/1
  Fcn5/1 -> Mux1/3
  Fcn4/1 -> Mux1/2
  Fcn3/1 -> Mux1/1
  u/1 -> Fcn5/1, Fcn4/1, Fcn3/1, Fcn2/1, Fcn1/1, Fcn/1

== system myLibrary/SG/Exciter/Exciter ST4B/Fex ==
  V_E : Inport
  Ifd : Inport  Port=2
  Data Type Conversion Inherited : simulink/Signal Attributes/Data Type Conversion Inherited  ConvertRealWorld=Real World Value  DoSatur=off
  Divide : Product  Inputs=*/
  Gain : Gain  Gain=K_C  OutDataTypeStr=double
  Prevent divide by zero : Fcn  Expr=u+(u==0)*eps
  fex : MATLAB Function  TreatAsAtomicUnit=on
  F_EX : Outport  VectorParamsAs1DForOutWhenUnconnected=off
  wires:
  Data Type Conversion Inherited/1 -> F_EX/1
  fex/1(F_EX) -> Data Type Conversion Inherited/2  "F_EX"
  Gain/1 -> fex/1(I_N)  "I_N"
  Divide/1 -> Gain/1
  V_E/1 -> Prevent divide by zero/1
  Ifd/1 -> Divide/1, Data Type Conversion Inherited/1
  Prevent divide by zero/1 -> Divide/2

== system myLibrary/SG/Exciter/Exciter ST4B/PI_M ==
  u : Inport
  Constant2 : Constant  Value=0
  Gain2 : Gain  Gain=K_PM
  Gain3 : Gain  Gain=K_IM
  Integrator (Discrete or Continuous) : eeGeneralControl/Integrator (Discrete or Continuous)  LabelModeActiveChoice=Discrete  ExternalReset=level  LimitType=Anti-windup  B=inf  A=-inf  Ts=Ts
  Sum6 : Sum
  y : Outport
  wires:
  Gain3/1 -> Integrator (Discrete or Continuous)/1, Integrator (Discrete or Continuous)/3
  u/1 -> Gain2/1, Gain3/1
  Constant2/1 -> Integrator (Discrete or Continuous)/2
  Integrator (Discrete or Continuous)/1 -> Sum6/2
  Gain2/1 -> Sum6/1
  Sum6/1 -> y/1

== system myLibrary/SG/Exciter/Exciter ST4B/PI_R ==
  u : Inport
  Constant2 : Constant  Value=0
  Gain2 : Gain  Gain=K_PR
  Gain3 : Gain  Gain=K_IR
  Integrator (Discrete or Continuous) : eeGeneralControl/Integrator (Discrete or Continuous)  LabelModeActiveChoice=Discrete  ExternalReset=level  LimitType=Anti-windup  B=inf  A=-inf  Ts=Ts
  Sum6 : Sum
  y : Outport
  wires:
  Gain3/1 -> Integrator (Discrete or Continuous)/1, Integrator (Discrete or Continuous)/3
  u/1 -> Gain2/1, Gain3/1
  Constant2/1 -> Integrator (Discrete or Continuous)/2
  Integrator (Discrete or Continuous)/1 -> Sum6/2
  Gain2/1 -> Sum6/1
  Sum6/1 -> y/1

== system myLibrary/SG/Exciter/Exciter ST4B/Subsystem1 ==
  V_T : Inport
  Gain1 : Gain  Gain=K_P
  Sqrt : Sqrt
  y : Outport
  wires:
  Gain1/1 -> Sqrt/1
  Sqrt/1 -> y/1
  V_T/1 -> Gain1/1

== system myLibrary/SG/Governor-Turbine/Steam Turbine and Governor/Model ==
  Pref : Inport
  wref : Inport  Port=2
  d_theta : Inport  Port=3
  wm : Inport  Port=4
  4 mass shaft : Subsystem  TreatAsAtomicUnit=on
  Constant3 : Constant  Value=T_SG.genType ~= 1
  Product : Product  InputSameDT=on  SaturateOnIntegerOverflow=on  OutDataTypeStr=Inherit: Same as first input
  Sum : Sum  Inputs=+  InputSameDT=on  SaturateOnIntegerOverflow=on  OutDataTypeStr=Inherit: Same as first input
  Switch1 : Switch  Threshold=0.5  SaturateOnIntegerOverflow=off
  Terminator1 : Terminator
  governor : Subsystem  mask(Speed regulator for thermal turbine){Rp=reg1(2)}
      mask prompts: Rp "Permanent droop Rp:"
  multi-mass : Constant  Value=T_SG.genType == 1
  steam turbine MM : Subsystem  mask(Thermal turbine){Fa=FA, Ta=turb1, f0=q0}
      mask prompts: Fa "Generator 1 torque fractions [ F1  F2  F3  F4 ]:"; Ta "Time constants [ T1  T2  T3  T4 ] (s):"; f0 "Initial flows f0:"
      mask init:
      | F2=Fa(1); F3=Fa(2); F4=Fa(3); F5=Fa(4);
      | if Ta(1)==0, T1=1; else T1=Ta(1); end; if Ta(2)==0, T2=1; else T2=Ta(2); end
      | if Ta(3)==0, T3=1; else T3=Ta(3); end; if Ta(4)==0, T4=1; else T4=Ta(4); end
  steam turbine SM : Subsystem  mask(Thermal turbine){Fa=FA, Ta=turb1, f0=q0}
      mask prompts: Fa "Generator 1 torque fractions [ F1  F2  F3  F4 ]:"; Ta "Time constants [ T1  T2  T3  T4 ] (s):"; f0 "Initial flows f0:"
      mask init:
      | F2=Fa(1); F3=Fa(2); F4=Fa(3); F5=Fa(4);
      | if Ta(1)==0, T1=1; else T1=Ta(1); end; if Ta(2)==0, T2=1; else T2=Ta(2); end
      | if Ta(3)==0, T3=1; else T3=Ta(3); end; if Ta(4)==0, T4=1; else T4=Ta(4); end
  Pm : Outport
  Tr5-2 : Outport  Port=2
  dw_5-2 : Outport  Port=3
  gate : Outport  Port=4
  wires:
  steam turbine SM/1(Tturb) -> Sum/1
  steam turbine MM/2(T5-2) -> 4 mass shaft/1(T5-2)
  governor/1(gate opening) -> gate/1, steam turbine MM/1(gate), steam turbine SM/1(gate)
  steam turbine MM/1(flowHp) -> Terminator1/1
  4 mass shaft/3(dw_5-2) -> dw_5-2/1
  d_theta/1 -> 4 mass shaft/2(d_theta)
  Constant3/1 -> Switch1/2
  Sum/1 -> Switch1/1
  4 mass shaft/1(Tm_g) -> Switch1/3
  Switch1/1 -> Product/1
  4 mass shaft/2(Tr2-5) -> Tr5-2/1
  Product/1 -> Pm/1
  wref/1 -> governor/2(wref)
  Pref/1 -> governor/1(Pref)
  wm/1 -> Product/2, governor/3(w)
  multi-mass/1 -> 4 mass shaft/Enable

== system myLibrary/SG_step/Exciter/Exciter ST4B/Fex ==
  V_E : Inport
  Ifd : Inport  Port=2
  Data Type Conversion Inherited : simulink/Signal Attributes/Data Type Conversion Inherited  ConvertRealWorld=Real World Value  DoSatur=off
  Divide : Product  Inputs=*/
  Gain : Gain  Gain=K_C  OutDataTypeStr=double
  Prevent divide by zero : Fcn  Expr=u+(u==0)*eps
  fex : MATLAB Function  TreatAsAtomicUnit=on
  F_EX : Outport  VectorParamsAs1DForOutWhenUnconnected=off
  wires:
  Data Type Conversion Inherited/1 -> F_EX/1
  fex/1(F_EX) -> Data Type Conversion Inherited/2  "F_EX"
  Gain/1 -> fex/1(I_N)  "I_N"
  Divide/1 -> Gain/1
  V_E/1 -> Prevent divide by zero/1
  Ifd/1 -> Divide/1, Data Type Conversion Inherited/1
  Prevent divide by zero/1 -> Divide/2

== system myLibrary/SG_step/Exciter/Exciter ST4B/PI_M ==
  u : Inport
  Constant2 : Constant  Value=0
  Gain2 : Gain  Gain=K_PM
  Gain3 : Gain  Gain=K_IM
  Integrator (Discrete or Continuous) : eeGeneralControl/Integrator (Discrete or Continuous)  LabelModeActiveChoice=Discrete  ExternalReset=level  LimitType=Anti-windup  B=inf  A=-inf  Ts=Ts
  Sum6 : Sum
  y : Outport
  wires:
  Gain3/1 -> Integrator (Discrete or Continuous)/1, Integrator (Discrete or Continuous)/3
  u/1 -> Gain2/1, Gain3/1
  Constant2/1 -> Integrator (Discrete or Continuous)/2
  Integrator (Discrete or Continuous)/1 -> Sum6/2
  Gain2/1 -> Sum6/1
  Sum6/1 -> y/1

== system myLibrary/SG_step/Exciter/Exciter ST4B/PI_R ==
  u : Inport
  Constant2 : Constant  Value=0
  Gain2 : Gain  Gain=K_PR
  Gain3 : Gain  Gain=K_IR
  Integrator (Discrete or Continuous) : eeGeneralControl/Integrator (Discrete or Continuous)  LabelModeActiveChoice=Discrete  ExternalReset=level  LimitType=Anti-windup  B=inf  A=-inf  Ts=Ts
  Sum6 : Sum
  y : Outport
  wires:
  Gain3/1 -> Integrator (Discrete or Continuous)/1, Integrator (Discrete or Continuous)/3
  u/1 -> Gain2/1, Gain3/1
  Constant2/1 -> Integrator (Discrete or Continuous)/2
  Integrator (Discrete or Continuous)/1 -> Sum6/2
  Gain2/1 -> Sum6/1
  Sum6/1 -> y/1

== system myLibrary/SG_step/Exciter/Exciter ST4B/Subsystem1 ==
  V_T : Inport
  Gain1 : Gain  Gain=K_P
  Sqrt : Sqrt
  y : Outport
  wires:
  Gain1/1 -> Sqrt/1
  Sqrt/1 -> y/1
  V_T/1 -> Gain1/1

== system myLibrary/SG_step/Governor-Turbine/Steam Turbine and Governor/Model ==
  Pref : Inport
  wref : Inport  Port=2
  d_theta : Inport  Port=3
  wm : Inport  Port=4
  4 mass shaft : Subsystem  TreatAsAtomicUnit=on
  Constant3 : Constant  Value=T_SG.genType ~= 1
  Product : Product  InputSameDT=on  SaturateOnIntegerOverflow=on  OutDataTypeStr=Inherit: Same as first input
  Sum : Sum  Inputs=+  InputSameDT=on  SaturateOnIntegerOverflow=on  OutDataTypeStr=Inherit: Same as first input
  Switch1 : Switch  Threshold=0.5  SaturateOnIntegerOverflow=off
  Terminator1 : Terminator
  governor : Subsystem  mask(Speed regulator for thermal turbine){Rp=reg1(2)}
      mask prompts: Rp "Permanent droop Rp:"
  multi-mass : Constant  Value=T_SG.genType == 1
  steam turbine MM : Subsystem  mask(Thermal turbine){Fa=FA, Ta=turb1, f0=q0}
      mask prompts: Fa "Generator 1 torque fractions [ F1  F2  F3  F4 ]:"; Ta "Time constants [ T1  T2  T3  T4 ] (s):"; f0 "Initial flows f0:"
      mask init:
      | F2=Fa(1); F3=Fa(2); F4=Fa(3); F5=Fa(4);
      | if Ta(1)==0, T1=1; else T1=Ta(1); end; if Ta(2)==0, T2=1; else T2=Ta(2); end
      | if Ta(3)==0, T3=1; else T3=Ta(3); end; if Ta(4)==0, T4=1; else T4=Ta(4); end
  steam turbine SM : Subsystem  mask(Thermal turbine){Fa=FA, Ta=turb1, f0=q0}
      mask prompts: Fa "Generator 1 torque fractions [ F1  F2  F3  F4 ]:"; Ta "Time constants [ T1  T2  T3  T4 ] (s):"; f0 "Initial flows f0:"
      mask init:
      | F2=Fa(1); F3=Fa(2); F4=Fa(3); F5=Fa(4);
      | if Ta(1)==0, T1=1; else T1=Ta(1); end; if Ta(2)==0, T2=1; else T2=Ta(2); end
      | if Ta(3)==0, T3=1; else T3=Ta(3); end; if Ta(4)==0, T4=1; else T4=Ta(4); end
  Pm : Outport
  Tr5-2 : Outport  Port=2
  dw_5-2 : Outport  Port=3
  gate : Outport  Port=4
  wires:
  steam turbine SM/1(Tturb) -> Sum/1
  steam turbine MM/2(T5-2) -> 4 mass shaft/1(T5-2)
  governor/1(gate opening) -> gate/1, steam turbine MM/1(gate), steam turbine SM/1(gate)
  steam turbine MM/1(flowHp) -> Terminator1/1
  4 mass shaft/3(dw_5-2) -> dw_5-2/1
  d_theta/1 -> 4 mass shaft/2(d_theta)
  Constant3/1 -> Switch1/2
  Sum/1 -> Switch1/1
  4 mass shaft/1(Tm_g) -> Switch1/3
  Switch1/1 -> Product/1
  4 mass shaft/2(Tr2-5) -> Tr5-2/1
  Product/1 -> Pm/1
  wref/1 -> governor/2(wref)
  Pref/1 -> governor/1(Pref)
  wm/1 -> Product/2, governor/3(w)
  multi-mass/1 -> 4 mass shaft/Enable

== system myLibrary/STATCOM/Control/Is/Matriu T ==
  u : Inport
  Constant : Constant  Value=(2/3)*[1/2 1/2 1/2]
  Fcn : Fcn  Expr=(2/3)*cos(u)
  Fcn1 : Fcn  Expr=(2/3)*cos(u-(2*pi)/3)
  Fcn2 : Fcn  Expr=(2/3)*cos(u+(2*pi)/3)
  Fcn3 : Fcn  Expr=(2/3)*sin(u)
  Fcn4 : Fcn  Expr=(2/3)*sin(u-(2*pi)/3)
  Fcn5 : Fcn  Expr=(2/3)*sin(u+(2*pi)/3)
  Math Function : Math  Operator=transpose  SignedPower=on
  Matrix Concatenate : Concatenate  NumInputs=3  Mode=Multidimensional array  ConcatenateDimension=2
  Mux : Mux  Inputs=3
  Mux1 : Mux  Inputs=3
  Out1 : Outport  VectorParamsAs1DForOutWhenUnconnected=off
  wires:
  Math Function/1 -> Out1/1
  Matrix Concatenate/1 -> Math Function/1
  Mux1/1 -> Matrix Concatenate/2
  Fcn2/1 -> Mux/3
  Fcn1/1 -> Mux/2
  Fcn/1 -> Mux/1
  Constant/1 -> Matrix Concatenate/3
  Mux/1 -> Matrix Concatenate/1
  Fcn5/1 -> Mux1/3
  Fcn4/1 -> Mux1/2
  Fcn3/1 -> Mux1/1
  u/1 -> Fcn5/1, Fcn4/1, Fcn3/1, Fcn2/1, Fcn1/1, Fcn/1

== system myLibrary/STATCOM/Control/Is1/Matriu T ==
  u : Inport
  Constant : Constant  Value=(2/3)*[1/2 1/2 1/2]
  Fcn : Fcn  Expr=(2/3)*cos(u)
  Fcn1 : Fcn  Expr=(2/3)*cos(u-(2*pi)/3)
  Fcn2 : Fcn  Expr=(2/3)*cos(u+(2*pi)/3)
  Fcn3 : Fcn  Expr=(2/3)*sin(u)
  Fcn4 : Fcn  Expr=(2/3)*sin(u-(2*pi)/3)
  Fcn5 : Fcn  Expr=(2/3)*sin(u+(2*pi)/3)
  Math Function : Math  Operator=transpose  SignedPower=on
  Matrix Concatenate : Concatenate  NumInputs=3  Mode=Multidimensional array  ConcatenateDimension=2
  Mux : Mux  Inputs=3
  Mux1 : Mux  Inputs=3
  Out1 : Outport  VectorParamsAs1DForOutWhenUnconnected=off
  wires:
  u/1 -> Fcn/1, Fcn1/1, Fcn2/1, Fcn3/1, Fcn4/1, Fcn5/1
  Fcn3/1 -> Mux1/1
  Fcn4/1 -> Mux1/2
  Fcn5/1 -> Mux1/3
  Mux/1 -> Matrix Concatenate/1
  Constant/1 -> Matrix Concatenate/3
  Fcn/1 -> Mux/1
  Fcn1/1 -> Mux/2
  Fcn2/1 -> Mux/3
  Mux1/1 -> Matrix Concatenate/2
  Matrix Concatenate/1 -> Math Function/1
  Math Function/1 -> Out1/1

== system myLibrary/STATCOM/Control/Is3/Matriu T ==
  u : Inport
  Constant : Constant  Value=(2/3)*[1/2 1/2 1/2]
  Fcn : Fcn  Expr=(2/3)*cos(u)
  Fcn1 : Fcn  Expr=(2/3)*cos(u-(2*pi)/3)
  Fcn2 : Fcn  Expr=(2/3)*cos(u+(2*pi)/3)
  Fcn3 : Fcn  Expr=(2/3)*sin(u)
  Fcn4 : Fcn  Expr=(2/3)*sin(u-(2*pi)/3)
  Fcn5 : Fcn  Expr=(2/3)*sin(u+(2*pi)/3)
  Math Function : Math  Operator=transpose  SignedPower=on
  Matrix Concatenate : Concatenate  NumInputs=3  Mode=Multidimensional array  ConcatenateDimension=2
  Mux : Mux  Inputs=3
  Mux1 : Mux  Inputs=3
  Out1 : Outport  VectorParamsAs1DForOutWhenUnconnected=off
  wires:
  Math Function/1 -> Out1/1
  Matrix Concatenate/1 -> Math Function/1
  Mux1/1 -> Matrix Concatenate/2
  Fcn2/1 -> Mux/3
  Fcn1/1 -> Mux/2
  Fcn/1 -> Mux/1
  Constant/1 -> Matrix Concatenate/3
  Mux/1 -> Matrix Concatenate/1
  Fcn5/1 -> Mux1/3
  Fcn4/1 -> Mux1/2
  Fcn3/1 -> Mux1/1
  u/1 -> Fcn5/1, Fcn4/1, Fcn3/1, Fcn2/1, Fcn1/1, Fcn/1

== system myLibrary/STATCOM/Control/Is4/Matriu T ==
  u : Inport
  Constant : Constant  Value=(2/3)*[1/2 1/2 1/2]
  Fcn : Fcn  Expr=(2/3)*cos(u)
  Fcn1 : Fcn  Expr=(2/3)*cos(u-(2*pi)/3)
  Fcn2 : Fcn  Expr=(2/3)*cos(u+(2*pi)/3)
  Fcn3 : Fcn  Expr=(2/3)*sin(u)
  Fcn4 : Fcn  Expr=(2/3)*sin(u-(2*pi)/3)
  Fcn5 : Fcn  Expr=(2/3)*sin(u+(2*pi)/3)
  Math Function : Math  Operator=transpose  SignedPower=on
  Matrix Concatenate : Concatenate  NumInputs=3  Mode=Multidimensional array  ConcatenateDimension=2
  Mux : Mux  Inputs=3
  Mux1 : Mux  Inputs=3
  Out1 : Outport  VectorParamsAs1DForOutWhenUnconnected=off
  wires:
  u/1 -> Fcn/1, Fcn1/1, Fcn2/1, Fcn3/1, Fcn4/1, Fcn5/1
  Fcn3/1 -> Mux1/1
  Fcn4/1 -> Mux1/2
  Fcn5/1 -> Mux1/3
  Mux/1 -> Matrix Concatenate/1
  Constant/1 -> Matrix Concatenate/3
  Fcn/1 -> Mux/1
  Fcn1/1 -> Mux/2
  Fcn2/1 -> Mux/3
  Mux1/1 -> Matrix Concatenate/2
  Matrix Concatenate/1 -> Math Function/1
  Math Function/1 -> Out1/1

== system myLibrary/STATCOM/Control/Is5/Matriu T ==
  u : Inport
  Constant : Constant  Value=(2/3)*[1/2 1/2 1/2]
  Fcn : Fcn  Expr=(2/3)*cos(u)
  Fcn1 : Fcn  Expr=(2/3)*cos(u-(2*pi)/3)
  Fcn2 : Fcn  Expr=(2/3)*cos(u+(2*pi)/3)
  Fcn3 : Fcn  Expr=(2/3)*sin(u)
  Fcn4 : Fcn  Expr=(2/3)*sin(u-(2*pi)/3)
  Fcn5 : Fcn  Expr=(2/3)*sin(u+(2*pi)/3)
  Math Function : Math  Operator=transpose  SignedPower=on
  Matrix Concatenate : Concatenate  NumInputs=3  Mode=Multidimensional array  ConcatenateDimension=2
  Mux : Mux  Inputs=3
  Mux1 : Mux  Inputs=3
  Out1 : Outport  VectorParamsAs1DForOutWhenUnconnected=off
  wires:
  Math Function/1 -> Out1/1
  Matrix Concatenate/1 -> Math Function/1
  Mux1/1 -> Matrix Concatenate/2
  Fcn2/1 -> Mux/3
  Fcn1/1 -> Mux/2
  Fcn/1 -> Mux/1
  Constant/1 -> Matrix Concatenate/3
  Mux/1 -> Matrix Concatenate/1
  Fcn5/1 -> Mux1/3
  Fcn4/1 -> Mux1/2
  Fcn3/1 -> Mux1/1
  u/1 -> Fcn5/1, Fcn4/1, Fcn3/1, Fcn2/1, Fcn1/1, Fcn/1

== system myLibrary/STATCOM/Control/Is7/Matriu T ==
  u : Inport
  Constant : Constant  Value=(2/3)*[1/2 1/2 1/2]
  Fcn : Fcn  Expr=(2/3)*cos(u)
  Fcn1 : Fcn  Expr=(2/3)*cos(u-(2*pi)/3)
  Fcn2 : Fcn  Expr=(2/3)*cos(u+(2*pi)/3)
  Fcn3 : Fcn  Expr=(2/3)*sin(u)
  Fcn4 : Fcn  Expr=(2/3)*sin(u-(2*pi)/3)
  Fcn5 : Fcn  Expr=(2/3)*sin(u+(2*pi)/3)
  Math Function : Math  Operator=transpose  SignedPower=on
  Matrix Concatenate : Concatenate  NumInputs=3  Mode=Multidimensional array  ConcatenateDimension=2
  Mux : Mux  Inputs=3
  Mux1 : Mux  Inputs=3
  Out1 : Outport  VectorParamsAs1DForOutWhenUnconnected=off
  wires:
  u/1 -> Fcn/1, Fcn1/1, Fcn2/1, Fcn3/1, Fcn4/1, Fcn5/1
  Fcn3/1 -> Mux1/1
  Fcn4/1 -> Mux1/2
  Fcn5/1 -> Mux1/3
  Mux/1 -> Matrix Concatenate/1
  Constant/1 -> Matrix Concatenate/3
  Fcn/1 -> Mux/1
  Fcn1/1 -> Mux/2
  Fcn2/1 -> Mux/3
  Mux1/1 -> Matrix Concatenate/2
  Matrix Concatenate/1 -> Math Function/1
  Math Function/1 -> Out1/1

== system myLibrary/STATCOM/Control/PLL/Tpark ==
  Va : Inport
  Vb : Inport  Port=2
  Vc : Inport  Port=3
  u : Inport  Port=4
  Demux : Demux  Outputs=3
  Matriu T : Subsystem
  Mux : Mux  Inputs=3
      settings: DisplayOption=signals
  Product : Product  Multiplication=Matrix(*)
  Vq : Outport  VectorParamsAs1DForOutWhenUnconnected=off
  Vd : Outport  Port=2  VectorParamsAs1DForOutWhenUnconnected=off
  0 : Outport  Port=3  VectorParamsAs1DForOutWhenUnconnected=off
  wires:
  Va/1 -> Mux/1
  Vb/1 -> Mux/2
  Vc/1 -> Mux/3
  Product/1 -> Demux/1
  Demux/1 -> Vq/1
  Demux/2 -> Vd/1
  Demux/3 -> 0/1
  u/1 -> Matriu T/1(u)
  Mux/1 -> Product/2
  Matriu T/1(Out1) -> Product/1

== system myLibrary/GFOL/Control/PLL/Tpark/Matriu T ==
  u : Inport
  Constant : Constant  Value=(2/3)*[1/2 1/2 1/2]
  Fcn : Fcn  Expr=(2/3)*cos(u)
  Fcn1 : Fcn  Expr=(2/3)*cos(u-(2*pi)/3)
  Fcn2 : Fcn  Expr=(2/3)*cos(u+(2*pi)/3)
  Fcn3 : Fcn  Expr=(2/3)*sin(u)
  Fcn4 : Fcn  Expr=(2/3)*sin(u-(2*pi)/3)
  Fcn5 : Fcn  Expr=(2/3)*sin(u+(2*pi)/3)
  Math Function : Math  Operator=transpose  SignedPower=on
  Matrix Concatenate : Concatenate  NumInputs=3  Mode=Multidimensional array  ConcatenateDimension=2
  Mux : Mux  Inputs=3
  Mux1 : Mux  Inputs=3
  Out1 : Outport  VectorParamsAs1DForOutWhenUnconnected=off
  wires:
  Math Function/1 -> Out1/1
  Matrix Concatenate/1 -> Math Function/1
  Mux1/1 -> Matrix Concatenate/2
  Fcn2/1 -> Mux/3
  Fcn1/1 -> Mux/2
  Fcn/1 -> Mux/1
  Constant/1 -> Matrix Concatenate/3
  Mux/1 -> Matrix Concatenate/1
  Fcn5/1 -> Mux1/3
  Fcn4/1 -> Mux1/2
  Fcn3/1 -> Mux1/1
  u/1 -> Fcn/1, Fcn1/1, Fcn2/1, Fcn3/1, Fcn4/1, Fcn5/1

== system myLibrary/GFOL_RL/Control/PLL/Tpark/Matriu T ==
  u : Inport
  Constant : Constant  Value=(2/3)*[1/2 1/2 1/2]
  Fcn : Fcn  Expr=(2/3)*cos(u)
  Fcn1 : Fcn  Expr=(2/3)*cos(u-(2*pi)/3)
  Fcn2 : Fcn  Expr=(2/3)*cos(u+(2*pi)/3)
  Fcn3 : Fcn  Expr=(2/3)*sin(u)
  Fcn4 : Fcn  Expr=(2/3)*sin(u-(2*pi)/3)
  Fcn5 : Fcn  Expr=(2/3)*sin(u+(2*pi)/3)
  Math Function : Math  Operator=transpose  SignedPower=on
  Matrix Concatenate : Concatenate  NumInputs=3  Mode=Multidimensional array  ConcatenateDimension=2
  Mux : Mux  Inputs=3
  Mux1 : Mux  Inputs=3
  Out1 : Outport  VectorParamsAs1DForOutWhenUnconnected=off
  wires:
  Math Function/1 -> Out1/1
  Matrix Concatenate/1 -> Math Function/1
  Mux1/1 -> Matrix Concatenate/2
  Fcn2/1 -> Mux/3
  Fcn1/1 -> Mux/2
  Fcn/1 -> Mux/1
  Constant/1 -> Matrix Concatenate/3
  Mux/1 -> Matrix Concatenate/1
  Fcn5/1 -> Mux1/3
  Fcn4/1 -> Mux1/2
  Fcn3/1 -> Mux1/1
  u/1 -> Fcn/1, Fcn1/1, Fcn2/1, Fcn3/1, Fcn4/1, Fcn5/1

== system myLibrary/SG/Governor-Turbine/Steam Turbine and Governor/Model/4 mass shaft ==
  T5-2 : Inport
  d_theta : Inport  Port=2
  Enable : EnablePort  PropagateVarSize=During execution
  1 mass : Subsystem  TreatAsAtomicUnit=on
  2 masses : Subsystem  TreatAsAtomicUnit=on
  3 masses : Subsystem  TreatAsAtomicUnit=on
  4 masses : Subsystem  TreatAsAtomicUnit=on
  Multiport Switch1 : MultiPortSwitch  Inputs=4  SaturateOnIntegerOverflow=off
  Multiport Switch2 : MultiPortSwitch  Inputs=4  SaturateOnIntegerOverflow=off
  Multiport Switch3 : MultiPortSwitch  Inputs=4  SaturateOnIntegerOverflow=off
  ctrl2 : Constant  Value=ctrl1==4
  ctrl3 : Constant  Value=ctrl1==3
  ctrl4 : Constant  Value=ctrl1
  ctrl6 : Constant  Value=ctrl1==2
  ctrl7 : Constant  Value=ctrl1==1
  Tm_g : Outport  OutputWhenDisabled=reset  InitialOutput=0
  Tr2-5 : Outport  Port=2  OutputWhenDisabled=reset  InitialOutput=[0 0 0 0]
  dw_5-2 : Outport  Port=3  OutputWhenDisabled=reset  InitialOutput=[0 0 0 0]
  wires:
  4 masses/2(dw_5-2) -> Multiport Switch3/5
  Multiport Switch3/1 -> dw_5-2/1
  Multiport Switch2/1 -> Tm_g/1
  Multiport Switch1/1 -> Tr2-5/1
  3 masses/2(dw_5-2) -> Multiport Switch3/4
  ctrl6/1 -> 2 masses/Enable
  ctrl7/1 -> 1 mass/Enable
  2 masses/2(dw_5-2) -> Multiport Switch3/3
  1 mass/2(dw_5-2) -> Multiport Switch3/2
  ctrl3/1 -> 3 masses/Enable
  ctrl2/1 -> 4 masses/Enable
  4 masses/3(Tm_gen) -> Multiport Switch2/5
  3 masses/3(Tm_gen) -> Multiport Switch2/4
  2 masses/3(Tm_gen) -> Multiport Switch2/3
  ctrl4/1 -> Multiport Switch3/1, Multiport Switch2/1, Multiport Switch1/1
  1 mass/3(Tm_gen) -> Multiport Switch2/2
  d_theta/1 -> 4 masses/2(dth_gen), 3 masses/2(dth_gen), 2 masses/2(dth_gen), 1 mass/2(dth_gen)
  T5-2/1 -> 4 masses/1(Tt_5-2), 3 masses/1(Tt_5-2), 2 masses/1(Tt_5-2), 1 mass/1(Tt_5-2)
  4 masses/1(Ts_5-2) -> Multiport Switch1/5
  3 masses/1(Ts_5-2) -> Multiport Switch1/4
  2 masses/1(Ts_5-2) -> Multiport Switch1/3
  1 mass/1(Ts_5-2) -> Multiport Switch1/2

== system myLibrary/SG/Governor-Turbine/Steam Turbine and Governor/Model/governor ==
  Pref : Inport
  wref : Inport  Port=2
  w : Inport  Port=3
  Gain : Gain  Gain=1/Rp  SaturateOnIntegerOverflow=on  OutDataTypeStr=Inherit: Same as input  ParamDataTypeStr=Inherit: Same as input
  Gain4 : Gain  Gain=1/Rp  SaturateOnIntegerOverflow=on  OutDataTypeStr=Inherit: Same as input  ParamDataTypeStr=Inherit: Same as input
  Sum3 : Sum  Inputs=++-  InputSameDT=on  SaturateOnIntegerOverflow=on  OutDataTypeStr=Inherit: Same as first input
  gate opening : Outport
  wires:
  wref/1 -> Gain4/1
  Sum3/1 -> gate opening/1
  w/1 -> Gain/1
  Gain/1 -> Sum3/3
  Pref/1 -> Sum3/1
  Gain4/1 -> Sum3/2

== system myLibrary/SG/Governor-Turbine/Steam Turbine and Governor/Model/steam turbine MM ==
  gate : Inport
  Gain : Gain  Gain=F2  SaturateOnIntegerOverflow=on  OutDataTypeStr=Inherit: Same as input  ParamDataTypeStr=Inherit: Same as input
  Gain2 : Gain  Gain=F3  SaturateOnIntegerOverflow=on  OutDataTypeStr=Inherit: Same as input  ParamDataTypeStr=Inherit: Same as input
  Gain3 : Gain  Gain=F4  SaturateOnIntegerOverflow=on  OutDataTypeStr=Inherit: Same as input  ParamDataTypeStr=Inherit: Same as input
  Gain4 : Gain  Gain=F5  SaturateOnIntegerOverflow=on  OutDataTypeStr=Inherit: Same as input  ParamDataTypeStr=Inherit: Same as input
  Mux : Mux
  Scope : Scope  NumInputPorts=4
  Stage 1 : Subsystem
  "Stage 2 " : Subsystem
  Stage 3 : Subsystem
  Stage 4 : Subsystem
  flowHp : Outport
  T5-2 : Outport  Port=2
  wires:
  Stage 4/1(Out1) -> Gain4/1, Stage 3/1(In1), Scope/2, flowHp/1
  gate/1 -> Stage 4/1(In1), Scope/1
  Stage 3/1(Out1) -> Gain3/1, "Stage 2 "/1(In1), Scope/3
  Gain4/1 -> Mux/1
  Gain3/1 -> Mux/2
  Gain2/1 -> Mux/3
  Gain/1 -> Mux/4
  "Stage 2 "/1(Out1) -> Gain2/1, Stage 1/1(In1), Scope/4
  Stage 1/1(Out1) -> Gain/1
  Mux/1 -> T5-2/1

== system myLibrary/SG/Governor-Turbine/Steam Turbine and Governor/Model/steam turbine SM ==
  gate : Inport
  Gain : Gain  Gain=(1-initMachineBlocks{SGnum,13}(1))
  Gain1 : Gain  Gain=initMachineBlocks{SGnum,13}(1)
  Stage4 : spsFirstOrderFilterLib/First-Order Filter  FilterType=Lowpass  Tc=initMachineBlocks{SGnum,13}(2)  Ts=Ts  Initialize=on  Vac_Init=[0, 0, T_SG.fb]  Vdc_Init=(1-initMachineBlocks{SGnum,13}(1))*initSG.Pm  PlotResponse=off  FreqRange="[0,  200,  1]"
  Sum : Sum  Inputs=++|
  Tturb : Outport
  wires:
  Stage4/1 -> Sum/2
  Gain1/1 -> Sum/1
  Sum/1 -> Tturb/1
  Gain/1 -> Stage4/1
  gate/1 -> Gain/1, Gain1/1
